simulink subsystem "Charge_port"  (R2024b)
settings: Solver=VariableStepAuto  StartTime=0.0  StopTime=10.0  RelTol=1e-3
values from neighbouring files (symbols this model uses):
  Charge_rate = 12*60    (= 720)    [load_vars.m]
  Is_chargin = 1    [load_vars.m]
settings Model: Creator=CoffeElliot  LastModifiedBy=CoffeElliot

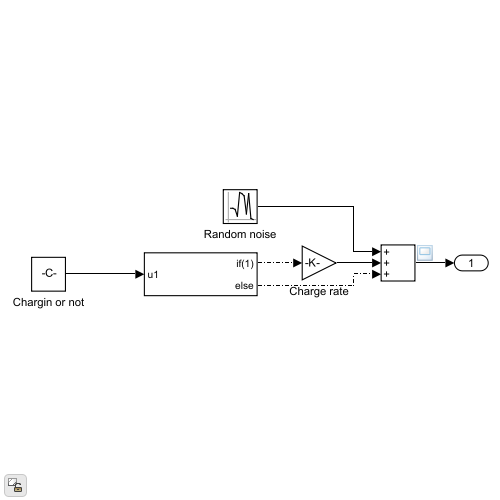
[thumbnail: Simulink's stored preview of the top-level diagram]
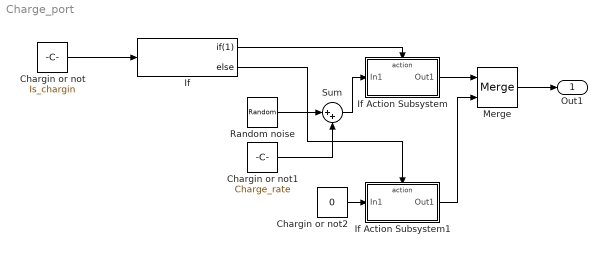
== system Charge_port ==
  Chargin or not : Constant  Value=Is_chargin  OutDataTypeStr=boolean
  Chargin or not1 : Constant  Value=Charge_rate  OutDataTypeStr=boolean
  Chargin or not2 : Constant  Value=0  OutDataTypeStr=boolean
  If : If  IfExpression=1
  If Action Subsystem : Subsystem  TreatAsAtomicUnit=on
  If Action Subsystem1 : Subsystem  TreatAsAtomicUnit=on
  Merge : Merge
  Random noise : RandomNumber  Variance=10  SampleTime=0.1
  Sum : Sum  Inputs=|++
  Out1 : Outport
  wires:
  Chargin or not/1 -> If/1
  Chargin or not1/1 -> Sum/2
  If/2 -> If Action Subsystem1/Action
  Merge/1 -> Out1/1
  Random noise/1 -> Sum/1
  Sum/1 -> If Action Subsystem/1(In1)
  If/1 -> If Action Subsystem/Action
  If Action Subsystem/1(Out1) -> Merge/1
  Chargin or not2/1 -> If Action Subsystem1/1(In1)
  If Action Subsystem1/1(Out1) -> Merge/2

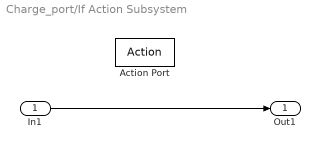
== system Charge_port/If Action Subsystem ==
  In1 : Inport
  Action Port : ActionPort
  Out1 : Outport
  wires:
  In1/1 -> Out1/1

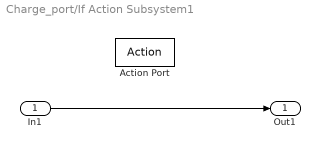
== system Charge_port/If Action Subsystem1 ==
  In1 : Inport
  Action Port : ActionPort
  Out1 : Outport
  wires:
  In1/1 -> Out1/1
